simulink model "Motor_Mixer_Test"  (R2017a)
settings: Solver=VariableStepAuto  StartTime=0.0  StopTime=10  RelTol=1e-3
undefined symbols (not defined in the file or in its folder): Ts
libraries: aerolibactuator x4
settings Model: Creator=GusBus  LastModifiedBy=GusBus

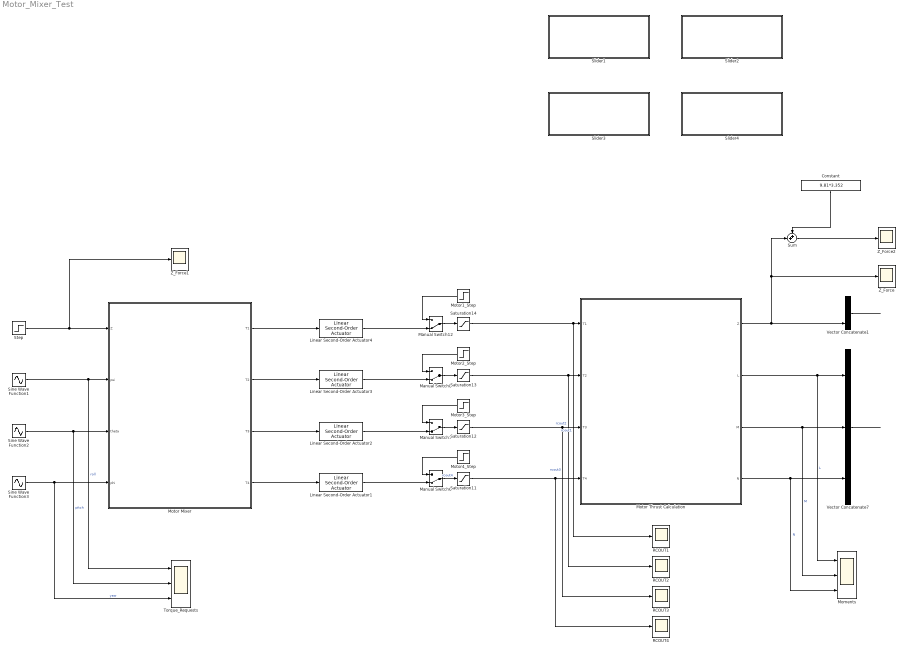
== system Motor_Mixer_Test ==
  Constant : Constant  Value=9.81*3.352
  Linear Second-Order Actuator{1..4} (4 alike) : aerolibactuator/Linear Second-Order Actuator  wn_fin=750  z_fin=1.5  fin_act_0=0  fin_act_vel=0
      settings: SourceProductName=Aerospace Blockset  SourceProductBaseCode=AE
  Manual Switch{6..8,12} (4 alike) : ManualSwitch  CurrentSetting=0
  Moments : Scope  NumInputPorts=3
  Motor Mixer : MATLAB Function  TreatAsAtomicUnit=on
  Motor Thrust Calculation : MATLAB Function  TreatAsAtomicUnit=on
  Motor1_Step : Step  Time=0.1  Before=1000  After=1365.671641791  SampleTime=0
  Motor2_Step : Step  Time=0.1  Before=1000  After=1855.223880597  SampleTime=0
  Motor3_Step : Step  Time=0.1  Before=1000  After=1368.6567164179  SampleTime=0
  Motor4_Step : Step  Time=0.1  Before=1000  After=1894.0298507463  SampleTime=0
  RCOUT{1..4} (4 alike) : Scope
  Saturation11 : Saturate  UpperLimit=-0.05  LowerLimit=-25
  Saturation12 : Saturate  UpperLimit=-0.05  LowerLimit=-25
  Saturation13 : Saturate  UpperLimit=-0.05  LowerLimit=-25
  Saturation14 : Saturate  UpperLimit=-0.025  LowerLimit=-25
  Sine Wave Function1 : Sin  SampleTime=Ts
  Sine Wave Function2 : Sin  Amplitude=0.75  SampleTime=Ts
  Sine Wave Function3 : Sin  Amplitude=0.5  SampleTime=Ts
  Slider1 : Subsystem  DialogController=hmiCreateDDGDialog  IsWebBlock=on  mask(MWDashboardBlock){webBlockId=0636af2c-d13b-4b12-a17b-0240a80ce0cc, webBlockType=slider, ShowInLibBrowser=on, ShowInitialText=on, HMISrcModelName=Motor_Mixer_Test}
      mask prompts: webBlockId "WebBlock Id"; webBlockType "WebBlock Type"; HMISrcModelName "Source Model"
      mask help: SimulinkHMI:dialogs:SliderDialogDesc
      mask Help: helpview([docroot '/mapfiles/simulink.map'], 'hmi_slider')
      mask Display:
      | if strcmp(get_param(bdroot(gcb),'BlockDiagramType'), 'library')
      |     image([(matlabroot) '/toolbox/simulink/hmi/icons/Slider.png']);
      | end
  Slider2 : Subsystem  DialogController=hmiCreateDDGDialog  IsWebBlock=on  mask(MWDashboardBlock){webBlockId=9520e207-98da-4771-9872-bbe086d58b48, webBlockType=slider, ShowInLibBrowser=on, ShowInitialText=on, HMISrcModelName=Motor_Mixer_Test}
      mask prompts: webBlockId "WebBlock Id"; webBlockType "WebBlock Type"; HMISrcModelName "Source Model"
      mask help: SimulinkHMI:dialogs:SliderDialogDesc
      mask Help: helpview([docroot '/mapfiles/simulink.map'], 'hmi_slider')
      mask Display:
      | if strcmp(get_param(bdroot(gcb),'BlockDiagramType'), 'library')
      |     image([(matlabroot) '/toolbox/simulink/hmi/icons/Slider.png']);
      | end
  Slider3 : Subsystem  DialogController=hmiCreateDDGDialog  IsWebBlock=on  mask(MWDashboardBlock){webBlockId=b9e98b27-6fcd-43bc-901f-6eb997191e33, webBlockType=slider, ShowInLibBrowser=on, ShowInitialText=on, HMISrcModelName=Motor_Mixer_Test}
      mask prompts: webBlockId "WebBlock Id"; webBlockType "WebBlock Type"; HMISrcModelName "Source Model"
      mask help: SimulinkHMI:dialogs:SliderDialogDesc
      mask Help: helpview([docroot '/mapfiles/simulink.map'], 'hmi_slider')
      mask Display:
      | if strcmp(get_param(bdroot(gcb),'BlockDiagramType'), 'library')
      |     image([(matlabroot) '/toolbox/simulink/hmi/icons/Slider.png']);
      | end
  Slider4 : Subsystem  DialogController=hmiCreateDDGDialog  IsWebBlock=on  mask(MWDashboardBlock){webBlockId=cce68117-2f9e-40a5-b647-a657cb9a88c9, webBlockType=slider, ShowInLibBrowser=on, ShowInitialText=on, HMISrcModelName=Motor_Mixer_Test}
      mask prompts: webBlockId "WebBlock Id"; webBlockType "WebBlock Type"; HMISrcModelName "Source Model"
      mask help: SimulinkHMI:dialogs:SliderDialogDesc
      mask Help: helpview([docroot '/mapfiles/simulink.map'], 'hmi_slider')
      mask Display:
      | if strcmp(get_param(bdroot(gcb),'BlockDiagramType'), 'library')
      |     image([(matlabroot) '/toolbox/simulink/hmi/icons/Slider.png']);
      | end
  Step : Step  Time=0.1  After=-40  SampleTime=0
  Sum : Sum  Inputs=++|
  Torque_Requests : Scope  NumInputPorts=3
  Vector Concatenate1 : Concatenate  NumInputs=3
  Vector Concatenate7 : Concatenate  NumInputs=3
  Z_Force : Scope
  Z_Force1 : Scope
  Z_Force2 : Scope
  wires:
  Saturation12/1 -> RCOUT3/1, Motor Thrust Calculation/3(T3)  "rcout3"
  Manual Switch8/1 -> Saturation13/1
  Saturation14/1 -> RCOUT1/1, Motor Thrust Calculation/1(T1)  "rcout1"
  Motor3_Step/1 -> Manual Switch7/1
  Motor1_Step/1 -> Manual Switch12/1
  Saturation13/1 -> RCOUT2/1, Motor Thrust Calculation/2(T2)  "rcout2"
  Manual Switch12/1 -> Saturation14/1
  Manual Switch7/1 -> Saturation12/1
  Motor4_Step/1 -> Manual Switch6/1
  Saturation11/1 -> RCOUT4/1, Motor Thrust Calculation/4(T4)
  Motor Thrust Calculation/3(M) -> Moments/2, Vector Concatenate7/2  "M"
  Motor Thrust Calculation/2(L) -> Moments/1, Vector Concatenate7/1  "L"
  Vector Concatenate1/1 -> ?
  Vector Concatenate7/1 -> ?
  Motor Thrust Calculation/1(Z) -> Z_Force/1, Sum/2, Vector Concatenate1/3
  Manual Switch6/1 -> Saturation11/1  "rcout4"
  Motor2_Step/1 -> Manual Switch8/1
  Motor Thrust Calculation/4(N) -> Moments/3, Vector Concatenate7/3  "N"
  Constant/1 -> Sum/1
  Sum/1 -> Z_Force2/1
  Sine Wave Function3/1 -> Torque_Requests/3, Motor Mixer/4(phi)  "yaw"
  Step/1 -> Z_Force1/1, Motor Mixer/1(Z)
  Sine Wave Function2/1 -> Torque_Requests/2, Motor Mixer/3(theta)  "pitch"
  Sine Wave Function1/1 -> Torque_Requests/1, Motor Mixer/2(psi)  "roll"
  Motor Mixer/1(T1) -> Linear Second-Order Actuator4/1
  Motor Mixer/2(T2) -> Linear Second-Order Actuator3/1
  Motor Mixer/3(T3) -> Linear Second-Order Actuator2/1
  Motor Mixer/4(T4) -> Linear Second-Order Actuator1/1
  Linear Second-Order Actuator1/1 -> Manual Switch6/2
  Linear Second-Order Actuator2/1 -> Manual Switch7/2
  Linear Second-Order Actuator3/1 -> Manual Switch8/2
  Linear Second-Order Actuator4/1 -> Manual Switch12/2

== system Motor_Mixer_Test/Slider1 ==

== system Motor_Mixer_Test/Slider2 ==

== system Motor_Mixer_Test/Slider3 ==

== system Motor_Mixer_Test/Slider4 ==

== matlab function Motor_Mixer_Test/Motor Mixer ==
  data: Z input; T1 output; T2 output; psi input; T3 output; theta input; phi input; T4 output
function [T1,T2,T3,T4]  = fcn(Z, psi, theta, phi)
%       ccw       cw            
%N         3    1
%           \  /
%            \/
%            /\
%           /  \
%          2    4       
%       cw        ccw   E
%%%%%%%%%%%%%%%%%%%%%%%%%

%% Inputs
armLength           = 0.41;            %Meters
alpha               = deg2rad(15);     %Rad
chordLength         = 0.040;           %Meters
liftDragRatio       = 0.1;

roll_arm    = armLength * sin(alpha);
pitch_arm   = armLength * cos(alpha);
yaw_arm     = chordLength/liftDragRatio;
%% 

roll_contribution   = [-roll_arm roll_arm roll_arm -roll_arm];
pitch_contribution  = [pitch_arm -pitch_arm pitch_arm -pitch_arm];
yaw_contribution    = [-yaw_arm -yaw_arm yaw_arm yaw_arm];

contribution_matrix = [1 1 1 1; roll_contribution; pitch_contribution; yaw_contribution];

thrust_matrix = inv(contribution_matrix)*[Z;psi;theta;phi];

T1 = thrust_matrix(1,1);
T2 = thrust_matrix(2,1);
T3 = thrust_matrix(3,1);
T4 = thrust_matrix(4,1);

== matlab function Motor_Mixer_Test/Motor Thrust Calculation ==
  data: T1 input; Z output; T2 input; T3 input; T4 input; L output; M output; N output
function [Z, L, M, N]  = fcn(T1,T2,T3,T4)
%       ccw       cw            
%N         3    1
%           \  /
%            \/
%            /\
%           /  \
%          2    4       
%       cw        ccw   E
%%%%%%%%%%%%%%%%%%%%%%%%%

%% Inputs
armLength           = 0.41;            %Meters
alpha               = deg2rad(15);     %Rad
chordLength         = 0.040;           %Meters
liftDragRatio       = 0.1;

roll_arm    = armLength * sin(alpha);
pitch_arm   = armLength * cos(alpha);
yaw_arm     = chordLength/liftDragRatio;
%% 

roll_contribution   = [-roll_arm roll_arm roll_arm -roll_arm];
pitch_contribution  = [pitch_arm -pitch_arm pitch_arm -pitch_arm];
yaw_contribution    = [-yaw_arm -yaw_arm yaw_arm yaw_arm];

contribution_matrix = [1 1 1 1; roll_contribution; pitch_contribution; yaw_contribution];

moment_matrix = (contribution_matrix)*[T1;T2;T3;T4];

Z = moment_matrix(1,1);
L = moment_matrix(2,1);
M = moment_matrix(3,1);
N = moment_matrix(4,1);
